simulink model "a0_px4demo_PositionAndRateController"  (R2023b)
settings: Solver=FixedStepAuto  StartTime=0.0  StopTime=inf  FixedStep=0.004  RelTol=1e-3  EnableMultiTasking=on
PreLoadFcn:
  | if ispc
  | SampleTime = 0.01
  | PID_x_P = 0.8580043859649122
  | PID_x_I = 0
  | PID_x_D = 0.3097345132743363
  | PID_x_N = 10
  | 
  | PID_vx_P = 9.961622807017545
  | PID_vx_I = 0
  | PID_vx_D = 0.1081612586037365
  | PID_vx_N = 10
  | 
  | PID_y_P = 0.85
  | PID_y_I = 0
  | PID_y_D = 0.3
  | PID_y_N = 10
  | 
  | PID_vy_P = 10
  | PID_vy_I = 0
  | PID_vy_D = 0.1
  | PID_vy_N = 10
  | 
  | PID_z_P = 2.001693480101609
  | PID_z_I = 0.1
  | PID_z_D = 0.5
  | PID_z_N = 10
  | 
  | PID_vz_P = 1.906858594411516
  | PID_vz_I = 0.1
  | PID_vz_D = 0.09829059829059829
  | PID_vz_N = 10
  | 
  | PID_yaw_P = 0.08024000000000001
  | PID_yaw_I = 0.005
  | PID_yaw_D = 0.075
  | PID_yaw_N = 100
  | 
  | elseif isunix
  | SampleTime = 0.004
  | PID_x_P = 0.6
  | PID_x_I = 0
  | PID_x_D = 0.15
  | PID_x_N = 1
  | 
  | PID_vx_P = 8
  | PID_vx_I = 0
  | PID_vx_D = 0.05
  | PID_vx_N = 1
  | 
  | PID_y_P = 0.6
  | PID_y_I = 0
  | PID_y_D = 0.15
  | PID_y_N = 1
  | 
  | PID_vy_P = 8
  | PID_vy_I = 0
  | PID_vy_D = 0.05
  | PID_vy_N = 1
  | 
  | PID_z_P = 1.5
  | PID_z_I = 0.1
  | PID_z_D = 0.2
  | PID_z_N = 1
  | 
  | PID_vz_P = 1.5
  | PID_vz_I = 0.1
  | PID_vz_D = 0.05
  | PID_vz_N = 1
  | 
  | PID_yaw_P = 0.06
  | PID_yaw_I = 0.005
  | PID_yaw_D = 0.07
  | PID_yaw_N = 50
  | 
  | end
undefined symbols (not defined in the file or in its folder): dev, Main, pwm_output0
libraries: slpidlib x9, px4uORBlib x4, simulink_extras x3, sharedTrackingLibrary x2, sharedtransform x1, px4lib x1
(part 1 of 2)
CloseFcn:
  | clear PID_yaw*;
  | clear PID_x*;
  | clear PID_vx*;
  | clear PID_y*;
  | clear PID_vy*;
  | clear PID_z*;
  | clear PID_vz*;
  | clear SampleTime;
settings Model: ExtModeTrigDuration=3001  Creator=The MathWorks, Inc.  LastModifiedBy=uav2
settings SolverCC: AlgebraicLoopSolver=TrustRegion  PositivePriorityOrder=on  MaxZcPerStep=1
settings OptimizationCC: EnhancedBackFolding=on  PassReuseOutputArgsAs=Individual arguments  ZeroExternalMemoryAtStartup=off  ZeroInternalMemoryAtStartup=off  MaxStackSize=64  OptimizeBlockOrder=speed  DifferentSizesBufferReuse=on  OptimizationCustomize=off  EfficientTunableParamExpr=on
settings DebuggingCC: ParameterTunabilityLossMsg=error  UnconnectedInputMsg=warning  UnconnectedOutputMsg=warning  UnconnectedLineMsg=warning  SubsystemReferenceDiagnosticForUnitTest=warning
settings HardwareCC: ProdBitPerPointer=32  ProdBitPerSizeT=32  ProdBitPerPtrDiffT=32  ProdLargestAtomicInteger=Long  ProdLargestAtomicFloat=Double  ProdWordSize=32  ProdLongLongMode=on  ProdHWDeviceType=ARM Compatible->ARM Cortex
settings ModelReferenceCC: EnableRefExpFcnMdlSchedulingChecks=on
settings SFSimCC: MATLABDynamicMemAlloc=off  SimTargetLang=C++
settings RTWCC: Description=Embedded Coder  SystemTargetFile=ert.tlc  HardwareBoard=PX4 Host Target  TLCOptions="-aInlineSetEventsForThisBaseRateFcn=TLC_FALSE -aSuppressMultiTaskScheduler=TLC_FALSE  -aRateBasedStepFcn=0"  TemplateMakefile=ert_default_tmf  Toolchain=GNU Tools for PX4 Autopilots  PortableWordSizes=on  TargetLang=C++  DLArmComputeVersion=19.05
settings CodeAppCC: ForceParamTrailComments=on  IgnoreCustomStorageClasses=off  OperatorAnnotations=on  SimulinkDataObjDesc=on  SFDataObjDesc=on  InsertBlockDesc=on
settings ERTTargetCC: ExtModeTransport=2  ExtModeStaticAlloc=on  ExtModeMexFile=ext_xcp  ExtModeIntrfLevel=Level2 - Open

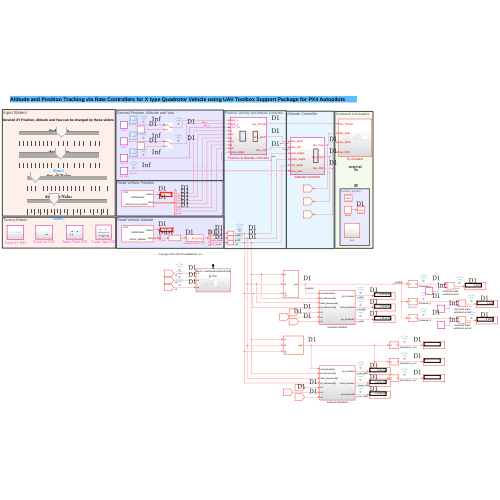
[thumbnail: Simulink's stored preview of the top-level diagram]
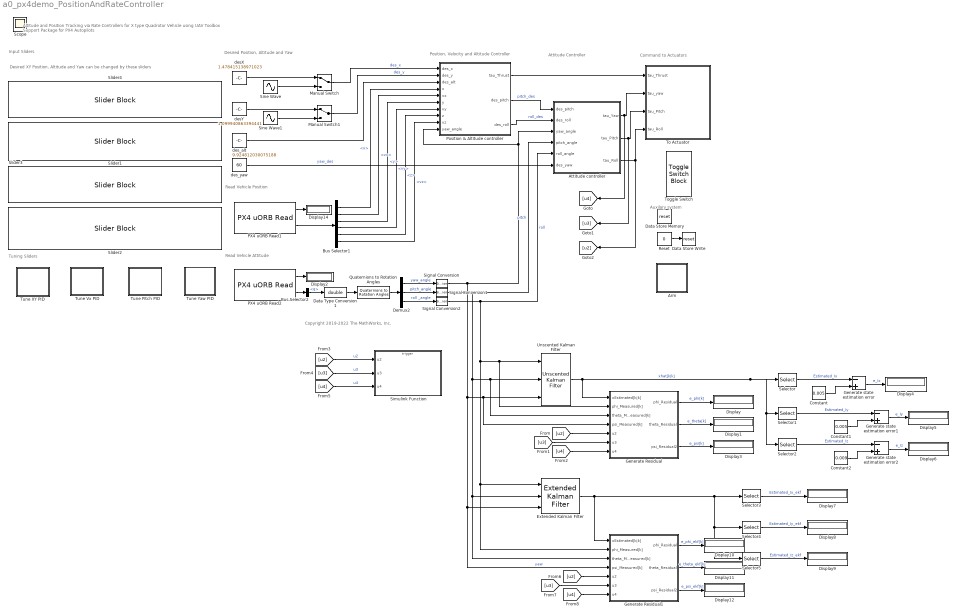
== system a0_px4demo_PositionAndRateController ==
  note: Input Sliders
  note: Command to Actuators
  note: Tuning Sliders
  note: Attitude Controller
  note: Desired Position, Altitude and Yaw
  note: Position, Velocity and Altitude Controller
  note: Read Vehicle Attitude
  note: Read Vehicle Position
  note: Auxilary system
  note: Altitude and Position Tracking via Rate Controllers for X type Quadrotor Vehicle using UAV Toolbox Support Package for PX4 Autopilots
  note: Copyright 2019-2022 The MathWorks, Inc.
  note: Desired XY Position, Altitude and Yaw can be changed by these sliders
  Arm : Subsystem
  Attitude controller : Subsystem
  Bus Selector1 : BusSelector  OutputSignals=x,vx,y,vy,z,vz
  Bus Selector2 : BusSelector  OutputSignals=q
  Constant : Constant  Value=0.005
  Constant1 : Constant  Value=0.005
  Constant2 : Constant  Value=0.009
  Data Store Write : DataStoreWrite  DataStoreName=reset  IndexOptions=Index vector (dialog)  Indices=1  OutputSizes=1
  Data Store Memory : DataStoreMemory  DataStoreName=reset  ReadBeforeWriteMsg=warning  WriteAfterWriteMsg=warning  WriteAfterReadMsg=warning  ShowAdditionalParam=off  OutDataTypeStr=boolean
  Data Type Conversion1 : DataTypeConversion  OutDataTypeStr=double  SaturateOnIntegerOverflow=off  RndMeth=Floor
  Demux2 : Demux  Outputs=3
  Display{,1..12,14} (14 alike) : Display
  Extended Kalman Filter : sharedTrackingLibrary/Extended Kalman Filter  StateTransitionFcn=uavStateFcnSimulink  HasStateTransitionJacobianFcn=off  HasAdditiveProcessNoise=Additive  ProcessNoise=0.00001  HasTimeVaryingProcessNoise=off  HasStateTransitionFcnExtraArgument=0  InitialState=[0;0;0;0;0;0;0;0;0;0.003;0.003;0.003]  InitialStateCovariance=0.00001  MeasurementFcn1=uavMeasurementFcn1  HasMeasurementJacobianFcn1=off  HasMeasurementEnablePort1=off  HasAdditiveMeasurementNoise1=Additive  MeasurementNoise1=0.00001  HasTimeVaryingMeasurementNoise1=off  HasMeasurementFcnExtraArgument1=0  HasMeasurementWrapping1=off  MeasurementFcn2=uavMeasurementFcn2  HasMeasurementJacobianFcn2=off  HasMeasurementEnablePort2=off  HasAdditiveMeasurementNoise2=Additive  MeasurementNoise2=0.00001  HasTimeVaryingMeasurementNoise2=off  HasMeasurementFcnExtraArgument2=0  HasMeasurementWrapping2=off  MeasurementFcn3=uavMeasurementFcn3  HasMeasurementJacobianFcn3=off  HasMeasurementEnablePort3=off  HasAdditiveMeasurementNoise3=Additive  MeasurementNoise3=0.00001  HasTimeVaryingMeasurementNoise3=off  HasMeasurementFcnExtraArgument3=0  HasMeasurementWrapping3=off  MeasurementFcn4=myMeasurementFcn  HasMeasurementJacobianFcn4=off  HasMeasurementEnablePort4=off  HasAdditiveMeasurementNoise4=Additive  MeasurementNoise4=1  HasTimeVaryingMeasurementNoise4=off  HasMeasurementFcnExtraArgument4=0  HasMeasurementWrapping4=off  MeasurementFcn5=myMeasurementFcn  HasMeasurementJacobianFcn5=off  HasMeasurementEnablePort5=off  HasAdditiveMeasurementNoise5=Additive  MeasurementNoise5=1  HasTimeVaryingMeasurementNoise5=off  HasMeasurementFcnExtraArgument5=0  HasMeasurementWrapping5=off  EnableMultirate=off  StateTransitionFcnSampleTime=1  MeasurementFcn1SampleTime=1  MeasurementFcn2SampleTime=1  MeasurementFcn3SampleTime=1  MeasurementFcn4SampleTime=1  MeasurementFcn5SampleTime=1  UseCurrentEstimator=on  OutputStateCovariance=off  DataType=double  SampleTime=0.004  NumberOfMeasurements=3
  Generate Residual : Subsystem
  Generate Residual1 : Subsystem
  Generate state estimation error : Sum  Inputs=-+
  Generate state estimation error1 : Sum  Inputs=-+
  Generate state estimation error2 : Sum  Inputs=-+
  Manual Switch : ManualSwitch
  Manual Switch1 : ManualSwitch
  PX4 uORB Read1 : px4uORBlib/PX4 uORB Read  uORBTopic=vehicle_local_position  selectInstance=vehicle_local_position_groundtruth  SampleTime=-1  BlockingMode=off  BlockTimeout=1e-3
  PX4 uORB Read2 : px4uORBlib/PX4 uORB Read  uORBTopic=vehicle_attitude  selectInstance=vehicle_attitude_groundtruth  SampleTime=0.004  BlockingMode=off  BlockTimeout=1e-3
  Position & Altitude controller : Subsystem
  Quaternions to Rotation Angles : sharedtransform/Quaternions to Rotation Angles  rotationOrder=ZYX  aMode=aMode
  Reset : Constant  Value=0  OutDataTypeStr=boolean  SampleTime=-1
      settings: OpenFcn=|
      | if strcmp('0',get_param(gcb, 'Value'))                        set_param(gcb, 'Value', '1');
      | else
      |             set_param(gcb, 'Value', '0');
      | end
  Selector : Selector  InputPortWidth=12  IndexOptions=Index vector (dialog)  Indices=10  OutputSizes=1
  Selector1 : Selector  InputPortWidth=12  IndexOptions=Index vector (dialog)  Indices=11  OutputSizes=1
  Selector2 : Selector  InputPortWidth=12  IndexOptions=Index vector (dialog)  Indices=12  OutputSizes=1
  Selector3 : Selector  InputPortWidth=12  IndexOptions=Index vector (dialog)  Indices=10  OutputSizes=1
  Selector4 : Selector  InputPortWidth=12  IndexOptions=Index vector (dialog)  Indices=11  OutputSizes=1
  Selector5 : Selector  InputPortWidth=12  IndexOptions=Index vector (dialog)  Indices=12  OutputSizes=1
  Signal Conversion : SignalConversion  OverrideOpt=off
  Signal Conversion1 : SignalConversion  OverrideOpt=off
  Signal Conversion2 : SignalConversion  OverrideOpt=off
  Simulink Function : Subsystem  TreatAsAtomicUnit=on
  Sine Wave : Sin  Amplitude=10  Frequency=2*pi*0.08
  Sine Wave1 : Sin  Amplitude=10  Frequency=2*pi*0.08  Phase=pi/2
  Slider1 : SliderBlock  ScaleMin=-20  ScaleMax=20
  Slider2 : SliderBlock  ScaleMax=180
  Slider3 : SliderBlock
  Slider4 : SliderBlock  ScaleMin=-20  ScaleMax=20
  To Actuator : Subsystem
  Toggle Switch : ToggleSwitchBlock
      settings: Values={{'Off', 'On'}, [0 1]}
  Tune Pitch PID : Subsystem
  Tune Vx PID : Subsystem
  Tune XY PID : Subsystem
  Tune Yaw PID : Subsystem
  Unscented Kalman Filter : sharedTrackingLibrary/Unscented Kalman Filter  StateTransitionFcn=uavStateFcnSimulink  HasAdditiveProcessNoise=Additive  ProcessNoise=0.00001  HasTimeVaryingProcessNoise=off  HasStateTransitionFcnExtraArgument=0  InitialState=[0;0;0;0;0;0;0;0;0;0.003;0.003;0.003]  InitialStateCovariance=0.00001  Alpha=1e-3  Beta=2  Kappa=0  MeasurementFcn1=uavMeasurementFcn1  HasMeasurementEnablePort1=off  HasAdditiveMeasurementNoise1=Additive  MeasurementNoise1=0.00001  HasTimeVaryingMeasurementNoise1=off  HasMeasurementFcnExtraArgument1=0  HasMeasurementWrapping1=off  MeasurementFcn2=uavMeasurementFcn2  HasMeasurementEnablePort2=off  HasAdditiveMeasurementNoise2=Additive  MeasurementNoise2=0.00001  HasTimeVaryingMeasurementNoise2=off  HasMeasurementFcnExtraArgument2=0  HasMeasurementWrapping2=off  MeasurementFcn3=uavMeasurementFcn3  HasMeasurementEnablePort3=off  HasAdditiveMeasurementNoise3=Additive  MeasurementNoise3=0.00001  HasTimeVaryingMeasurementNoise3=off  HasMeasurementFcnExtraArgument3=0  HasMeasurementWrapping3=off  MeasurementFcn4=uavMeasurementFcn4  HasMeasurementEnablePort4=off  HasAdditiveMeasurementNoise4=Nonadditive  MeasurementNoise4=1  HasTimeVaryingMeasurementNoise4=off  HasMeasurementFcnExtraArgument4=0  HasMeasurementWrapping4=off  MeasurementFcn5=uavMeasurementFcn5  HasMeasurementEnablePort5=off  HasAdditiveMeasurementNoise5=Nonadditive  MeasurementNoise5=1  HasTimeVaryingMeasurementNoise5=off  HasMeasurementFcnExtraArgument5=0  HasMeasurementWrapping5=off  EnableMultirate=off  StateTransitionFcnSampleTime=1  MeasurementFcn1SampleTime=1  MeasurementFcn2SampleTime=1  MeasurementFcn3SampleTime=1  MeasurementFcn4SampleTime=1  MeasurementFcn5SampleTime=1  UseCurrentEstimator=on  OutputStateCovariance=off  DataType=double  SampleTime=0.004  NumberOfMeasurements=3
  desX : Constant  Value=1.478415138971023
  desY : Constant  Value=1.099940863394441
  des_alt : Constant  Value=9.924812030075188
  des_yaw : Constant  Value=60
  Scope : Scope
  wires:
  Position & Altitude controller/1(tau_Thrust) -> To Actuator/1(tau_Thrust)
  Demux2/2 -> Signal Conversion1/1  "pitch_angle"
  Attitude controller/3(tau_Roll) -> To Actuator/4(tau_Roll), [u2]
  Bus Selector1/6 -> Position & Altitude controller/9(vz)  "<vz>"
  Bus Selector1/2 -> Position & Altitude controller/5(vx)  "<vx>"
  Bus Selector2/1 -> Data Type Conversion1/1  "<q>"
  PX4 uORB Read2/1 -> Display2/1
  Demux2/3 -> Signal Conversion2/1  "roll _angle"
  Sine Wave1/1 -> Manual Switch1/2
  PX4 uORB Read1/1 -> Display14/1
  Manual Switch1/1 -> Position & Altitude controller/2(des_y)  "des_y"
  Demux2/1 -> Signal Conversion/1  "yaw_angle"
  Manual Switch/1 -> Position & Altitude controller/1(des_x)  "des_x"
  Bus Selector1/5 -> Position & Altitude controller/8(z)  "<z>"
  Bus Selector1/4 -> Position & Altitude controller/7(vy)  "<vy>"
  PX4 uORB Read1/2 -> Bus Selector1/1
  PX4 uORB Read2/2 -> Bus Selector2/1
  Bus Selector1/1 -> Position & Altitude controller/4(x)  "<x>"
  des_yaw/1 -> Attitude controller/6(des_yaw)  "yaw_des"
  Data Type Conversion1/1 -> Quaternions to Rotation Angles/1
  Quaternions to Rotation Angles/1 -> Demux2/1
  Reset/1 -> Data Store Write/1
  Bus Selector1/3 -> Position & Altitude controller/6(y)  "<y>"
  desX/1 -> Manual Switch/1
  Sine Wave/1 -> Manual Switch/2
  desY/1 -> Manual Switch1/1
  des_alt/1 -> Position & Altitude controller/3(des_alt)
  Attitude controller/1(tau_Yaw) -> [u4], To Actuator/2(tau_yaw)
  Attitude controller/2(tau_Pitch) -> [u3], To Actuator/3(tau_Pitch)
  Generate Residual/1(phi_Residual) -> Display/1  "e_phi[k]"
  Generate Residual/2(theta_Residual) -> Display1/1  "e_theta[k]"
  Generate Residual/3(psi_Residual2) -> Display3/1  "e_psi[k]"
  [u2] -> Generate Residual/5(u2)
  [u3] -> Generate Residual/6(u3)
  [u4] -> Generate Residual/7(u4)
  Generate state estimation error/1 -> Display4/1  "e_Ix"
  Selector/1 -> Generate state estimation error/1  "Estimated_Ix"
  Unscented Kalman Filter/1 -> Selector2/1, Selector1/1, Selector/1, Generate Residual/1(xEstimated[k|k])  "xhat[k|k]"
  Constant/1 -> Generate state estimation error/2
  [u3] -> Simulink Function/2(u3)  "u3"
  [u2] -> Simulink Function/1(u2)  "u2"
  [u4] -> Simulink Function/3(u4)  "u4"
  Signal Conversion1/1 -> Generate Residual1/3(theta_Measured[k]), Extended Kalman Filter/2, Generate Residual/3(theta_Measured[k]), Unscented Kalman Filter/2, Attitude controller/4(pitch_angle)  "pitch"
  Signal Conversion2/1 -> Generate Residual1/2(phi_Measured[k]), Extended Kalman Filter/1, Generate Residual/2(phi_Measured[k]), Unscented Kalman Filter/1, Attitude controller/5("roll_angle ")  "roll"
  Selector1/1 -> Generate state estimation error1/1  "Estimated_Iy"
  Selector2/1 -> Generate state estimation error2/1  "Estimated_Iz"
  Constant1/1 -> Generate state estimation error1/2
  Generate state estimation error1/1 -> Display5/1  "e_Iy"
  Generate state estimation error2/1 -> Display6/1  "e_Iz"
  Constant2/1 -> Generate state estimation error2/2
  Position & Altitude controller/2(des_pitch) -> Attitude controller/1(des_pitch)  "pitch_des"
  Position & Altitude controller/3(des_roll) -> Attitude controller/2(des_roll)  "roll_des"
  Signal Conversion/1 -> Attitude controller/3(yaw_angle), Position & Altitude controller/10(yaw_angle), Generate Residual1/4(psi_Measured[k]), Extended Kalman Filter/3, Generate Residual/4(psi_Measured[k]), Unscented Kalman Filter/3  "yaw"
  Extended Kalman Filter/1 -> Generate Residual1/1(xEstimated[k|k]), Selector5/1, Selector4/1, Selector3/1
  Selector3/1 -> Display7/1  "Estimated_Ix_ekf"
  Selector4/1 -> Display8/1  "Estimated_Iy_ekf"
  Selector5/1 -> Display9/1  "Estimated_Iz_ekf"
  [u2] -> Generate Residual1/5(u2)
  [u3] -> Generate Residual1/6(u3)
  [u4] -> Generate Residual1/7(u4)
  Generate Residual1/1(phi_Residual) -> Display10/1  "e_phi_ekf[k]"
  Generate Residual1/2(theta_Residual) -> Display11/1  "e_theta_ekf[k]"
  Generate Residual1/3(psi_Residual2) -> Display12/1  "e_psi_ekf[k]"

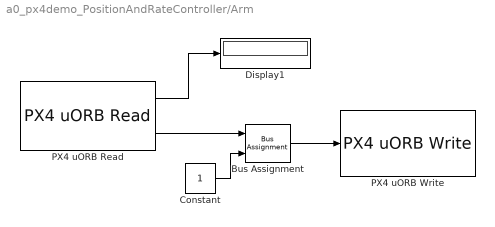
== system a0_px4demo_PositionAndRateController/Arm ==
  Bus Assignment : BusAssignment  AssignedSignals=armed
  Constant : Constant  OutDataTypeStr=Inherit: Inherit via back propagation  SampleTime=-1
  Display1 : Display
  PX4 uORB Read : px4uORBlib/PX4 uORB Read  uORBTopic=actuator_armed  selectInstance=actuator_armed  SampleTime=-1  BlockingMode=off  BlockTimeout=1e-3
  PX4 uORB Write : px4uORBlib/PX4 uORB Write  uORBTopic=actuator_armed  selectInstance=actuator_armed  MessageQueueLen=1
  wires:
  PX4 uORB Read/2 -> Bus Assignment/1
  PX4 uORB Read/1 -> Display1/1
  Bus Assignment/1 -> PX4 uORB Write/1
  Constant/1 -> Bus Assignment/2

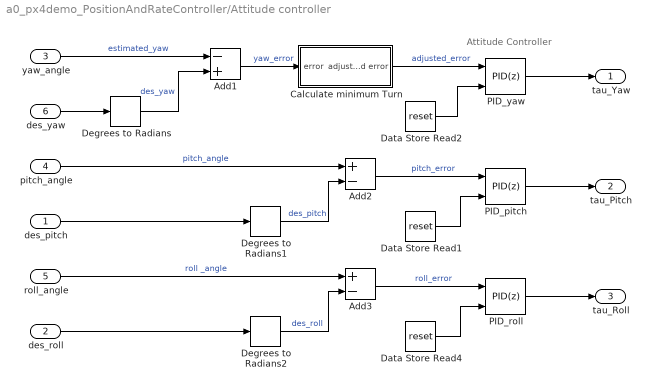
== system a0_px4demo_PositionAndRateController/Attitude controller ==
  note: Attitude Controller
  des_pitch : Inport
  des_roll : Inport  Port=2
  yaw_angle : Inport  Port=3
  pitch_angle : Inport  Port=4
  "roll_angle " : Inport  Port=5
  des_yaw : Inport  Port=6
  Add1 : Sum  Inputs=-+
  Add2 : Sum  Inputs=+-
  Add3 : Sum  Inputs=+-
  Calculate minimum Turn : Subsystem
  Data Store Read1 : DataStoreRead  DataStoreName=reset  IndexOptions=Index vector (dialog)  Indices=1  OutputSizes=1
  Data Store Read2 : DataStoreRead  DataStoreName=reset  IndexOptions=Index vector (dialog)  Indices=1  OutputSizes=1
  Data Store Read4 : DataStoreRead  DataStoreName=reset  IndexOptions=Index vector (dialog)  Indices=1  OutputSizes=1
  Degrees to Radians : simulink_extras/Transformations/Degrees to Radians
  Degrees to Radians1 : simulink_extras/Transformations/Degrees to Radians
  Degrees to Radians2 : simulink_extras/Transformations/Degrees to Radians
  PID_pitch : slpidlib/PID Controller  Controller=PID  Form=Parallel  TimeDomain=Discrete-time  UseExternalTs=off  SampleTime=-1  IntegratorMethod=Backward Euler  FilterMethod=Forward Euler  ControllerParametersSource=internal  P=0.027  I=0.005  UseKiTs=off  D=0.0145948093220339  N=50  UseFilter=on  TunerSelectOption=Transfer Function Based (PID Tuner App)  InitialConditionSource=internal  InitialConditionForIntegrator=0  InitialConditionForFilter=0  DifferentiatorICPrevScaledInput=0  ExternalReset=level  TrackingMode=off  Kt=1  LimitOutput=on  SatLimitsSource=internal  UpperSaturationLimit=0.05  LowerSaturationLimit=-0.05  LinearizeAsGain=off  AntiWindupMode=none  Kb=1  LimitIntegrator=off  UpperIntegratorSaturationLimit=inf  LowerIntegratorSaturationLimit=-inf  POutMin=[]  POutMax=[]  IOutMin=[]  IOutMax=[]  DOutMin=[]  DOutMax=[]  NOutMin=[]  NOutMax=[]  SumOutMin=[]  SumOutMax=[]  SaturationOutMin=[]  SaturationOutMax=[]  PParamMin=[]  PParamMax=[]  IParamMin=[]  IParamMax=[]  DParamMin=[]  DParamMax=[]  NParamMin=[]  NParamMax=[]  KbParamMin=[]  KbParamMax=[]  KtParamMin=[]  KtParamMax=[]  KbOutMin=[]  KbOutMax=[]  KtOutMin=[]  KtOutMax=[]  IntegratorOutMin=[]  IntegratorOutMax=[]  FilterOutMin=[]  FilterOutMax=[]  SumI1OutMin=[]  SumI1OutMax=[]  SumI2OutMin=[]  SumI2OutMax=[]  SumI3OutMin=[]  SumI3OutMax=[]  SumI4OutMin=[]  SumI4OutMax=[]  SumDOutMin=[]  SumDOutMax=[]  DifferentiatorOutMin=[]  DifferentiatorOutMax=[]  FilterDiffOutCoefMin=[]  FilterDiffOutCoefMax=[]  ReciprocalOutMin=[]  ReciprocalOutMax=[]  SumDenOutMin=[]  SumDenOutMax=[]  SumNumOutMin=[]  SumNumOutMax=[]  DivideOutMin=[]  DivideOutMax=[]  UdiffTsProdOutMin=[]  UdiffTsProdOutMax=[]  NTsProdOutMin=[]  NTsProdOutMax=[]  UintegralTsProdOutMin=[]  UintegralTsProdOutMax=[]  UngainTsProdOutMin=[]  UngainTsProdOutMax=[]  ClampingZeroOutDataTypeStr=Inherit: Inherit via back propagation  ClampingZeroOutMin=[]  ClampingZeroOutMax=[]  FilterDenConstantOutDataTypeStr=Inherit: Inherit via back propagation  FilterDenConstantOutMin=[]  FilterDenConstantOutMax=[]  PCopyOutDataTypeStr=Inherit: Inherit via back propagation  PCopyOutMin=[]  PCopyOutMax=[]  NCopyOutDataTypeStr=Inherit: Inherit via back propagation  NCopyOutMin=[]  NCopyOutMax=[]  IntegratorContinuousStateAttributes=''  IntegratorStateMustResolveToSignalObject=off  IntegratorRTWStateStorageClass=Auto  FilterContinuousStateAttributes=''  FilterStateMustResolveToSignalObject=off  FilterRTWStateStorageClass=Auto  ParallelPVariant=InternalParameters  IdealPVariant=Disabled  IVariant=InternalParameters  DVariant=InternalParameters  IntegratorVariant=Discrete  SatVariant=Enabled  AWVariant=Passthrough  PCopyVariant=Disabled  TRVariant=Disabled  FdbkBlocksVariant=Forward  IdealPFdbkVariant=Disabled  SatFdbkVariant=Disabled  DerivativeFilterVariant=ForwardEulerFilter  NVariant=InternalParameters  NCopyVariant=Disabled  FilterICVariant=InternalICsFilter  IntegratorICVariant=InternalICs  ExternalResetVariant=ExternalReset  TRSumVariant=Passthrough  SumFdbkVariant=Disabled  SumVariant=Sum_PID  TsampFilterVariant=InternalTs  TsampNgainVariant=Passthrough  TsampIntegralVariant=Disabled_SignalSpec  ExternalSaturationOutDataTypeStr=Inherit: Same as second input
  PID_roll : slpidlib/PID Controller  Controller=PID  Form=Parallel  TimeDomain=Discrete-time  UseExternalTs=off  SampleTime=-1  IntegratorMethod=Backward Euler  FilterMethod=Forward Euler  ControllerParametersSource=internal  P=0.03  I=0.005  UseKiTs=off  D=0.015  N=100  UseFilter=on  TunerSelectOption=Transfer Function Based (PID Tuner App)  InitialConditionSource=internal  InitialConditionForIntegrator=0  InitialConditionForFilter=0  DifferentiatorICPrevScaledInput=0  ExternalReset=level  TrackingMode=off  Kt=1  LimitOutput=on  SatLimitsSource=internal  UpperSaturationLimit=0.05  LowerSaturationLimit=-0.05  LinearizeAsGain=off  AntiWindupMode=none  Kb=1  LimitIntegrator=off  UpperIntegratorSaturationLimit=inf  LowerIntegratorSaturationLimit=-inf  POutMin=[]  POutMax=[]  IOutMin=[]  IOutMax=[]  DOutMin=[]  DOutMax=[]  NOutMin=[]  NOutMax=[]  SumOutMin=[]  SumOutMax=[]  SaturationOutMin=[]  SaturationOutMax=[]  PParamMin=[]  PParamMax=[]  IParamMin=[]  IParamMax=[]  DParamMin=[]  DParamMax=[]  NParamMin=[]  NParamMax=[]  KbParamMin=[]  KbParamMax=[]  KtParamMin=[]  KtParamMax=[]  KbOutMin=[]  KbOutMax=[]  KtOutMin=[]  KtOutMax=[]  IntegratorOutMin=[]  IntegratorOutMax=[]  FilterOutMin=[]  FilterOutMax=[]  SumI1OutMin=[]  SumI1OutMax=[]  SumI2OutMin=[]  SumI2OutMax=[]  SumI3OutMin=[]  SumI3OutMax=[]  SumI4OutMin=[]  SumI4OutMax=[]  SumDOutMin=[]  SumDOutMax=[]  DifferentiatorOutMin=[]  DifferentiatorOutMax=[]  FilterDiffOutCoefMin=[]  FilterDiffOutCoefMax=[]  ReciprocalOutMin=[]  ReciprocalOutMax=[]  SumDenOutMin=[]  SumDenOutMax=[]  SumNumOutMin=[]  SumNumOutMax=[]  DivideOutMin=[]  DivideOutMax=[]  UdiffTsProdOutMin=[]  UdiffTsProdOutMax=[]  NTsProdOutMin=[]  NTsProdOutMax=[]  UintegralTsProdOutMin=[]  UintegralTsProdOutMax=[]  UngainTsProdOutMin=[]  UngainTsProdOutMax=[]  ClampingZeroOutDataTypeStr=Inherit: Inherit via back propagation  ClampingZeroOutMin=[]  ClampingZeroOutMax=[]  FilterDenConstantOutDataTypeStr=Inherit: Inherit via back propagation  FilterDenConstantOutMin=[]  FilterDenConstantOutMax=[]  PCopyOutDataTypeStr=Inherit: Inherit via back propagation  PCopyOutMin=[]  PCopyOutMax=[]  NCopyOutDataTypeStr=Inherit: Inherit via back propagation  NCopyOutMin=[]  NCopyOutMax=[]  IntegratorContinuousStateAttributes=''  IntegratorStateMustResolveToSignalObject=off  IntegratorRTWStateStorageClass=Auto  FilterContinuousStateAttributes=''  FilterStateMustResolveToSignalObject=off  FilterRTWStateStorageClass=Auto  ParallelPVariant=InternalParameters  IdealPVariant=Disabled  IVariant=InternalParameters  DVariant=InternalParameters  IntegratorVariant=Discrete  SatVariant=Enabled  AWVariant=Passthrough  PCopyVariant=Disabled  TRVariant=Disabled  FdbkBlocksVariant=Forward  IdealPFdbkVariant=Disabled  SatFdbkVariant=Disabled  DerivativeFilterVariant=ForwardEulerFilter  NVariant=InternalParameters  NCopyVariant=Disabled  FilterICVariant=InternalICsFilter  IntegratorICVariant=InternalICs  ExternalResetVariant=ExternalReset  TRSumVariant=Passthrough  SumFdbkVariant=Disabled  SumVariant=Sum_PID  TsampFilterVariant=InternalTs  TsampNgainVariant=Passthrough  TsampIntegralVariant=Disabled_SignalSpec  ExternalSaturationOutDataTypeStr=Inherit: Same as second input
  PID_yaw : slpidlib/PID Controller  Controller=PID  Form=Parallel  TimeDomain=Discrete-time  UseExternalTs=off  SampleTime=-1  IntegratorMethod=Backward Euler  FilterMethod=Forward Euler  ControllerParametersSource=internal  P=PID_yaw_P  I=PID_yaw_I  UseKiTs=off  D=PID_yaw_D  N=PID_yaw_N  UseFilter=on  TunerSelectOption=Transfer Function Based (PID Tuner App)  InitialConditionSource=internal  InitialConditionForIntegrator=0  InitialConditionForFilter=0  DifferentiatorICPrevScaledInput=0  ExternalReset=level  TrackingMode=off  Kt=1  LimitOutput=on  SatLimitsSource=internal  UpperSaturationLimit=0.1  LowerSaturationLimit=-0.1  LinearizeAsGain=off  AntiWindupMode=none  Kb=1  LimitIntegrator=off  UpperIntegratorSaturationLimit=inf  LowerIntegratorSaturationLimit=-inf  POutMin=[]  POutMax=[]  IOutMin=[]  IOutMax=[]  DOutMin=[]  DOutMax=[]  NOutMin=[]  NOutMax=[]  SumOutMin=[]  SumOutMax=[]  SaturationOutMin=[]  SaturationOutMax=[]  PParamMin=[]  PParamMax=[]  IParamMin=[]  IParamMax=[]  DParamMin=[]  DParamMax=[]  NParamMin=[]  NParamMax=[]  KbParamMin=[]  KbParamMax=[]  KtParamMin=[]  KtParamMax=[]  KbOutMin=[]  KbOutMax=[]  KtOutMin=[]  KtOutMax=[]  IntegratorOutMin=[]  IntegratorOutMax=[]  FilterOutMin=[]  FilterOutMax=[]  SumI1OutMin=[]  SumI1OutMax=[]  SumI2OutMin=[]  SumI2OutMax=[]  SumI3OutMin=[]  SumI3OutMax=[]  SumI4OutMin=[]  SumI4OutMax=[]  SumDOutMin=[]  SumDOutMax=[]  DifferentiatorOutMin=[]  DifferentiatorOutMax=[]  FilterDiffOutCoefMin=[]  FilterDiffOutCoefMax=[]  ReciprocalOutMin=[]  ReciprocalOutMax=[]  SumDenOutMin=[]  SumDenOutMax=[]  SumNumOutMin=[]  SumNumOutMax=[]  DivideOutMin=[]  DivideOutMax=[]  UdiffTsProdOutMin=[]  UdiffTsProdOutMax=[]  NTsProdOutMin=[]  NTsProdOutMax=[]  UintegralTsProdOutMin=[]  UintegralTsProdOutMax=[]  UngainTsProdOutMin=[]  UngainTsProdOutMax=[]  ClampingZeroOutDataTypeStr=Inherit: Inherit via back propagation  ClampingZeroOutMin=[]  ClampingZeroOutMax=[]  FilterDenConstantOutDataTypeStr=Inherit: Inherit via back propagation  FilterDenConstantOutMin=[]  FilterDenConstantOutMax=[]  PCopyOutDataTypeStr=Inherit: Inherit via back propagation  PCopyOutMin=[]  PCopyOutMax=[]  NCopyOutDataTypeStr=Inherit: Inherit via back propagation  NCopyOutMin=[]  NCopyOutMax=[]  IntegratorContinuousStateAttributes=''  IntegratorStateMustResolveToSignalObject=off  IntegratorRTWStateStorageClass=Auto  FilterContinuousStateAttributes=''  FilterStateMustResolveToSignalObject=off  FilterRTWStateStorageClass=Auto  ParallelPVariant=InternalParameters  IdealPVariant=Disabled  IVariant=InternalParameters  DVariant=InternalParameters  IntegratorVariant=Discrete  SatVariant=Enabled  AWVariant=Passthrough  PCopyVariant=Disabled  TRVariant=Disabled  FdbkBlocksVariant=Forward  IdealPFdbkVariant=Disabled  SatFdbkVariant=Disabled  DerivativeFilterVariant=ForwardEulerFilter  NVariant=InternalParameters  NCopyVariant=Disabled  FilterICVariant=InternalICsFilter  IntegratorICVariant=InternalICs  ExternalResetVariant=ExternalReset  TRSumVariant=Passthrough  SumFdbkVariant=Disabled  SumVariant=Sum_PID  TsampFilterVariant=InternalTs  TsampNgainVariant=Passthrough  TsampIntegralVariant=Disabled_SignalSpec  ExternalSaturationOutDataTypeStr=Inherit: Same as second input
  tau_Yaw : Outport
  tau_Pitch : Outport  Port=2
  tau_Roll : Outport  Port=3
  wires:
  PID_roll/1 -> tau_Roll/1
  Data Store Read4/1 -> PID_roll/2
  PID_pitch/1 -> tau_Pitch/1
  yaw_angle/1 -> Add1/1  "estimated_yaw"
  Data Store Read1/1 -> PID_pitch/2
  Add2/1 -> PID_pitch/1  "pitch_error"
  des_yaw/1 -> Degrees to Radians/1
  pitch_angle/1 -> Add2/1  "pitch_angle"
  Add3/1 -> PID_roll/1  "roll_error"
  Degrees to Radians/1 -> Add1/2  "des_yaw"
  PID_yaw/1 -> tau_Yaw/1
  Data Store Read2/1 -> PID_yaw/2
  Add1/1 -> Calculate minimum Turn/1(error)  "yaw_error"
  "roll_angle "/1 -> Add3/1  "roll _angle"
  des_roll/1 -> Degrees to Radians2/1
  Degrees to Radians1/1 -> Add2/2  "des_pitch"
  Degrees to Radians2/1 -> Add3/2  "des_roll"
  des_pitch/1 -> Degrees to Radians1/1
  Calculate minimum Turn/1(adjusted error) -> PID_yaw/1  "adjusted_error"

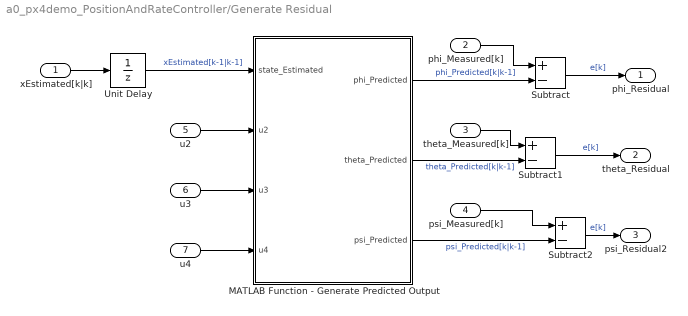
== system a0_px4demo_PositionAndRateController/Generate Residual ==
  xEstimated[k|k] : Inport
  phi_Measured[k] : Inport  Port=2
  theta_Measured[k] : Inport  Port=3
  psi_Measured[k] : Inport  Port=4
  u2 : Inport  Port=5
  u3 : Inport  Port=6
  u4 : Inport  Port=7
  MATLAB Function - Generate Predicted Output : MATLAB Function  TreatAsAtomicUnit=on
  Subtract : Sum  Inputs=+-
  Subtract1 : Sum  Inputs=+-
  Subtract2 : Sum  Inputs=+-
  Unit Delay : UnitDelay  InitialCondition=[0;0;0;0;0;0;0;0;0;0.003;0.003;0.003]  SampleTime=-1  HasFrameUpgradeWarning=on
  phi_Residual : Outport  VectorParamsAs1DForOutWhenUnconnected=off
  theta_Residual : Outport  Port=2  VectorParamsAs1DForOutWhenUnconnected=off
  psi_Residual2 : Outport  Port=3  VectorParamsAs1DForOutWhenUnconnected=off
  wires:
  xEstimated[k|k]/1 -> Unit Delay/1
  Unit Delay/1 -> MATLAB Function - Generate Predicted Output/1(state_Estimated)  "xEstimated[k-1|k-1]"
  MATLAB Function - Generate Predicted Output/1(phi_Predicted) -> Subtract/2  "phi_Predicted[k|k-1]"
  Subtract/1 -> phi_Residual/1  "e[k]"
  phi_Measured[k]/1 -> Subtract/1
  MATLAB Function - Generate Predicted Output/2(theta_Predicted) -> Subtract1/2  "theta_Predicted[k|k-1]"
  Subtract1/1 -> theta_Residual/1  "e[k]"
  MATLAB Function - Generate Predicted Output/3(psi_Predicted) -> Subtract2/2  "psi_Predicted[k|k-1]"
  Subtract2/1 -> psi_Residual2/1  "e[k]"
  theta_Measured[k]/1 -> Subtract1/1
  psi_Measured[k]/1 -> Subtract2/1
  u2/1 -> MATLAB Function - Generate Predicted Output/2(u2)
  u4/1 -> MATLAB Function - Generate Predicted Output/4(u4)
  u3/1 -> MATLAB Function - Generate Predicted Output/3(u3)

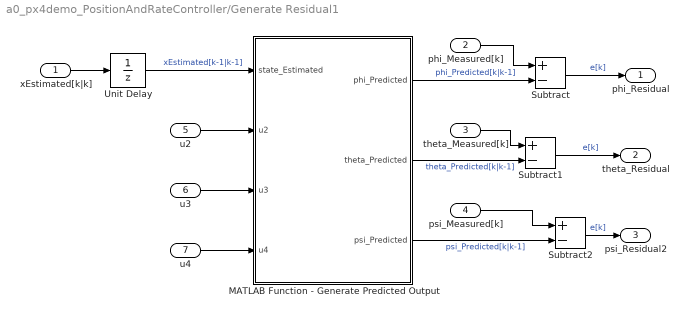
== system a0_px4demo_PositionAndRateController/Generate Residual1 ==
  xEstimated[k|k] : Inport
  phi_Measured[k] : Inport  Port=2
  theta_Measured[k] : Inport  Port=3
  psi_Measured[k] : Inport  Port=4
  u2 : Inport  Port=5
  u3 : Inport  Port=6
  u4 : Inport  Port=7
  MATLAB Function - Generate Predicted Output : MATLAB Function  TreatAsAtomicUnit=on
  Subtract : Sum  Inputs=+-
  Subtract1 : Sum  Inputs=+-
  Subtract2 : Sum  Inputs=+-
  Unit Delay : UnitDelay  InitialCondition=[0;0;0;0;0;0;0;0;0;0.003;0.003;0.003]  SampleTime=-1  HasFrameUpgradeWarning=on
  phi_Residual : Outport  VectorParamsAs1DForOutWhenUnconnected=off
  theta_Residual : Outport  Port=2  VectorParamsAs1DForOutWhenUnconnected=off
  psi_Residual2 : Outport  Port=3  VectorParamsAs1DForOutWhenUnconnected=off
  wires:
  u3/1 -> MATLAB Function - Generate Predicted Output/3(u3)
  u4/1 -> MATLAB Function - Generate Predicted Output/4(u4)
  u2/1 -> MATLAB Function - Generate Predicted Output/2(u2)
  psi_Measured[k]/1 -> Subtract2/1
  theta_Measured[k]/1 -> Subtract1/1
  Subtract2/1 -> psi_Residual2/1  "e[k]"
  MATLAB Function - Generate Predicted Output/3(psi_Predicted) -> Subtract2/2  "psi_Predicted[k|k-1]"
  Subtract1/1 -> theta_Residual/1  "e[k]"
  MATLAB Function - Generate Predicted Output/2(theta_Predicted) -> Subtract1/2  "theta_Predicted[k|k-1]"
  phi_Measured[k]/1 -> Subtract/1
  Subtract/1 -> phi_Residual/1  "e[k]"
  MATLAB Function - Generate Predicted Output/1(phi_Predicted) -> Subtract/2  "phi_Predicted[k|k-1]"
  Unit Delay/1 -> MATLAB Function - Generate Predicted Output/1(state_Estimated)  "xEstimated[k-1|k-1]"
  xEstimated[k|k]/1 -> Unit Delay/1
